simulink model "DroneDynamics_full"  (R2022b)
settings: Solver=VariableStepAuto  StartTime=0.0  StopTime=sim_time  FixedStep=dt  RelTol=1e-3
values from neighbouring files (symbols this model uses):
  b = 0.71    [Data_full.m]
  dt = 0.01    [Data_full.m]
  g_vect = [0; 0; m*g]    [Data_full.m]
  m = 3.074    [Data_full.m]
  mixer = [        -1         -1        -1         -1 ... (first row only)    [Data_full.m]
  NED2ECI = [ 1  0  0 ... (first row only)    [Data_full.m]
  omega0 = zeros(3,1)    [Data_full.m]
  p0 = zeros(3,1)    [Data_full.m]
  q0 = [1 0 0 0]'    [Data_full.m]
  tau = 1/900    (= 0.00111111111111)    [Data_full.m]
  v0 = zeros(3,1)    [Data_full.m]
undefined symbols (not defined in the file or in its folder): guidance
libraries: sharedtransform x1, simulink_extras x1, sim3dlib x1, uavsim3dlib x1
settings Model: Creator=Pietro Bruschi  LastModifiedBy=Utente
settings SFSimCC: SimCustomHeaderCode="#include \"controller_full.h\""  SimUserSources=controller_full.c  CustomCodeGlobalsAsFunctionIO=on

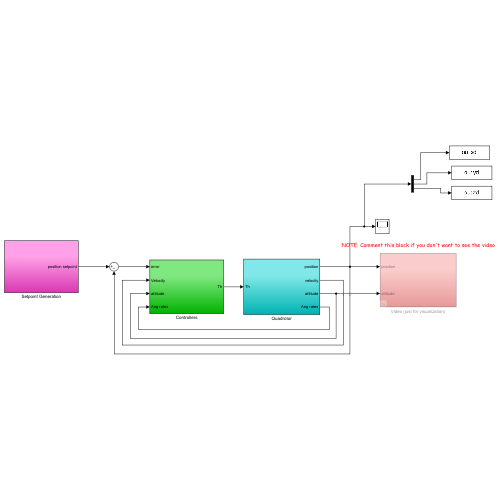
[thumbnail: Simulink's stored preview of the top-level diagram]
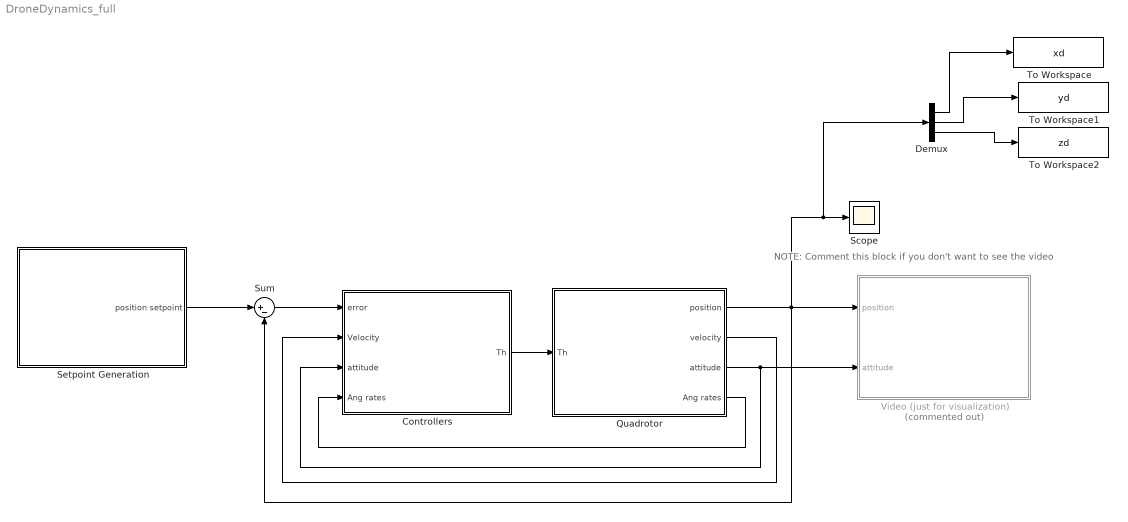
== system DroneDynamics_full ==
  note: NOTE: Comment this block if you don't want to see the video
  Controllers : Subsystem
  Demux : Demux  Outputs=3
  Quadrotor : Subsystem
  Scope : Scope
  Setpoint Generation : Subsystem
  Sum : Sum  Inputs=|+-
  To Workspace : ToWorkspace  VariableName=xd  SampleTime=-1
  To Workspace1 : ToWorkspace  VariableName=yd  SampleTime=-1
  To Workspace2 : ToWorkspace  VariableName=zd  SampleTime=-1
  Video (just for visualization) : Subsystem  Commented=on
  wires:
  Sum/1 -> Controllers/1("error ")
  Controllers/1(Th) -> Quadrotor/1(Th)
  Quadrotor/1(position) -> Demux/1, Scope/1, Sum/2, Video (just for visualization)/1(position)
  Setpoint Generation/1(position setpoint) -> Sum/1
  Quadrotor/4(Ang rates) -> Controllers/4(Ang rates)
  Quadrotor/3(attitude) -> Controllers/3(attitude), Video (just for visualization)/2(attitude)
  Quadrotor/2(velocity) -> Controllers/2(Velocity)
  Demux/1 -> To Workspace/1
  Demux/3 -> To Workspace2/1
  Demux/2 -> To Workspace1/1

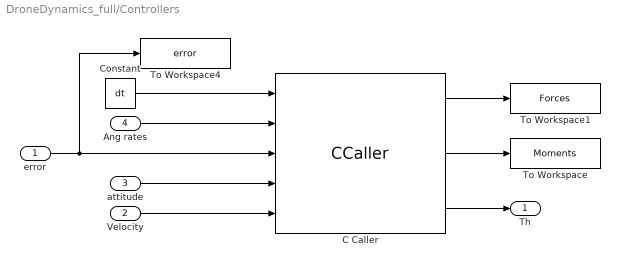
== system DroneDynamics_full/Controllers ==
  "error " : Inport
  Velocity : Inport  Port=2
  attitude : Inport  Port=3
  Ang rates : Inport  Port=4
  C Caller : CCaller  FunctionName=loop  PortSpecificationStruct="%)30     .    .!8   8    (     @         %    \"     T    !     0         %  0 \"0    $    _    07)G3F%M90  4&]R=$YA;64 4V-O<&4     26YD97@     5'EP90      4VEZ90      27-';&]B86P   X    X    !@    @    $          4    (     0    8    !         !     &    1%]L87-T   .    .     8    (    !          %    \"     $    &     0         0    !@   $1?;&%S=   #@   #@    &    \"     0         !0    @    !   ...(+7287 chars)"  SampleTime=dt
  Constant : Constant  Value=dt
  To Workspace : ToWorkspace  VariableName=Moments  SaveFormat=Timeseries  SampleTime=-1
  To Workspace1 : ToWorkspace  VariableName=Forces  SaveFormat=Timeseries  SampleTime=-1
  To Workspace4 : ToWorkspace  VariableName=error  SaveFormat=Timeseries  SampleTime=-1
  Th : Outport
  wires:
  "error "/1 -> To Workspace4/1, C Caller/3
  C Caller/1 -> To Workspace1/1
  C Caller/2 -> To Workspace/1
  C Caller/3 -> Th/1
  Velocity/1 -> C Caller/5
  attitude/1 -> C Caller/4
  Ang rates/1 -> C Caller/2
  Constant/1 -> C Caller/1

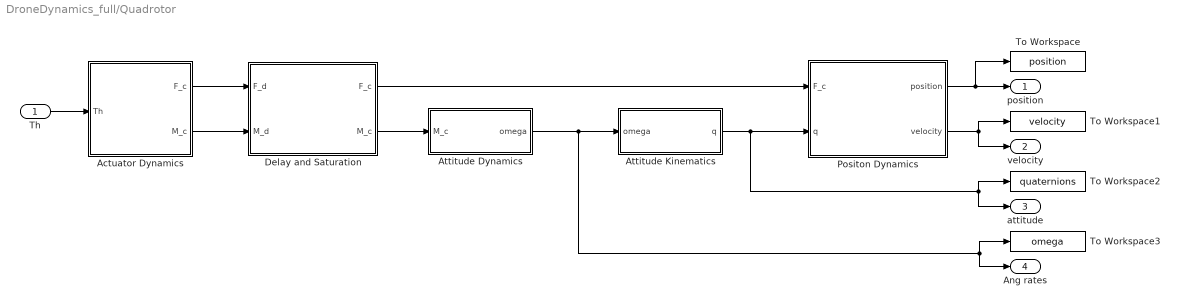
== system DroneDynamics_full/Quadrotor ==
  Th : Inport
  Actuator Dynamics : Subsystem
  Attitude Dynamics : Subsystem
  Attitude Kinematics : Subsystem
  Delay and Saturation : Subsystem
  Positon Dynamics : Subsystem
  To Workspace : ToWorkspace  VariableName=position  SaveFormat=Timeseries  SampleTime=-1
  To Workspace1 : ToWorkspace  VariableName=velocity  SaveFormat=Timeseries  SampleTime=-1
  To Workspace2 : ToWorkspace  VariableName=quaternions  SaveFormat=Timeseries  SampleTime=-1
  To Workspace3 : ToWorkspace  VariableName=omega  SaveFormat=Timeseries  SampleTime=-1
  position : Outport
  velocity : Outport  Port=2
  attitude : Outport  Port=3
  Ang rates : Outport  Port=4
  wires:
  Attitude Dynamics/1(omega) -> To Workspace3/1, Ang rates/1, Attitude Kinematics/1(omega)
  Attitude Kinematics/1(q) -> To Workspace2/1, attitude/1, Positon Dynamics/2(q)
  Positon Dynamics/1(position) -> To Workspace/1, position/1
  Positon Dynamics/2(velocity) -> velocity/1, To Workspace1/1
  Th/1 -> Actuator Dynamics/1(Th)
  Delay and Saturation/2(M_c) -> Attitude Dynamics/1(M_c)
  Actuator Dynamics/2(M_c) -> Delay and Saturation/2(M_d)
  Actuator Dynamics/1(F_c) -> Delay and Saturation/1(F_d)
  Delay and Saturation/1(F_c) -> Positon Dynamics/1(F_c)

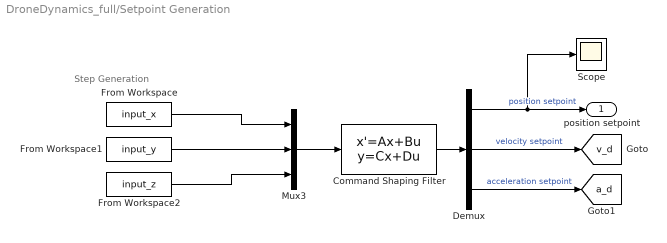
== system DroneDynamics_full/Setpoint Generation ==
  note: Step Generation
  "Command Shaping Filter " : StateSpace  A=guidance.A_d  B=guidance.B_d  C=eye(9)  D=zeros(9,3)  InitialCondition=zeros(9,1)  ParameterTunability=Unconstrained
  Demux : Demux  Outputs=3
  From Workspace : FromWorkspace  VariableName=input_x
  From Workspace1 : FromWorkspace  VariableName=input_y
  From Workspace2 : FromWorkspace  VariableName=input_z
  Mux3 : Mux  Inputs=3
  Scope : Scope
  position setpoint : Outport
  tag scope: a_d=global, v_d=global
  wires:
  "Command Shaping Filter "/1 -> Demux/1
  Mux3/1 -> "Command Shaping Filter "/1
  Demux/2 -> [v_d]  "velocity setpoint"
  Demux/3 -> [a_d]  "acceleration setpoint"
  Demux/1 -> Scope/1, position setpoint/1  "position setpoint"
  From Workspace/1 -> Mux3/1
  From Workspace1/1 -> Mux3/2
  From Workspace2/1 -> Mux3/3

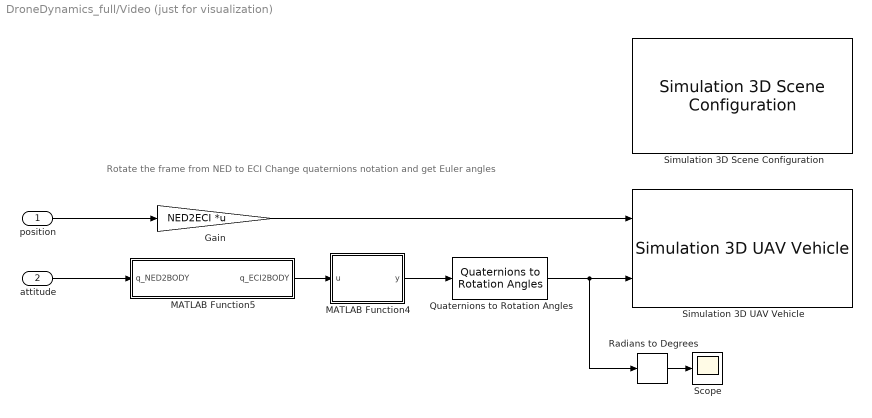
== system DroneDynamics_full/Video (just for visualization) ==
  note: Rotate the frame from NED to ECI
      | Change quaternions notation and get Euler angles
  position : Inport
  attitude : Inport  Port=2
  Gain : Gain  Gain=NED2ECI  Multiplication=Matrix(K*u)
  MATLAB Function4 : MATLAB Function  TreatAsAtomicUnit=on
  MATLAB Function5 : MATLAB Function  TreatAsAtomicUnit=on
  Quaternions to Rotation Angles : sharedtransform/Quaternions to Rotation Angles  rotationOrder=ZYX  aMode=aMode
  Radians to Degrees : simulink_extras/Transformations/Radians to Degrees
  Scope : Scope
  Simulation 3D Scene Configuration : sim3dlib/Simulation 3D Scene Configuration  Priority=0  ProjectFormat=Default Scenes  SceneDesc=US city block  ProjectName=C:\Program Files\MATLAB\R2022b\toolbox\shared\sim3d_projects\automotive_project\UE4\WindowsNoEditor\VehicleSimulation.exe  ScenePath=/Game/Maps/USCityBlock  EnableOpenDRIVE=off  vehTagList={'Scene Origin';'SimulinkVehicle1'}  vehTag=Scene Origin  OpVisEn=off  Ts=0.01  EnableWindow=on  EnableRemoteAccess=off  EnableWeather=off  SunAltitude=40.0  SunAzimuth=90  clouds=10  wind=1  fog=0  rain=0  EnableGeospatial=off  OriginHeight=200  OriginLatitude=40.744652  OriginLongitude=-73.988864  MapStyle=Aerial  AdditionalAssetIDs=[]  UseAdvancedSunSky=off  SolarTime=11  TimeZone=-5  Day=21  Month=9  Year=2022  UseDaylightSavingTime=on  DSTStartDay=10  DSTStartMonth=3  DSTEndDay=3  DSTEndMonth=11  DSTSwitchHour=2  sensorTag=MainCamera1  sensorId=1  sensorName=MainCamera1  mountLoc=Origin  offsetFlag=off  tmountOffset=[0, 0, 0]  rmountOffset=[0, 0, 0]  HorizontalResolution=1280  VerticalResolution=720  HorizontalFOV=60  mountPoint=[0 0 0]  mountOrientation=[0 0 0]  aMode=4  ID=1  GeoTrigger=Inactive
      settings: LibrarySourceBlock=uavsim3dlib/Simulation 3D Scene Configuration
  Simulation 3D UAV Vehicle : uavsim3dlib/Simulation 3D UAV Vehicle  Priority=-1  Mesh=Quadrotor  MeshPath=/MathWorksUAVContent/UAVs/HexaRotorUAV/HexaRotor.HexaRotor  Color=Black  ActorName=SimulinkVehicle1  InitialTranslation=[0 0 .2]  InitialRotation=[0 0 0]  SampleTime=-1  ActorType=SimulinkVehicle  ID=1  aMode=4  ActorTag=SimulinkVehicle1
  wires:
  Radians to Degrees/1 -> Scope/1
  MATLAB Function5/1(q_ECI2BODY) -> MATLAB Function4/1(u)
  position/1 -> Gain/1
  MATLAB Function4/1(y) -> Quaternions to Rotation Angles/1
  Gain/1 -> Simulation 3D UAV Vehicle/1
  attitude/1 -> MATLAB Function5/1(q_NED2BODY)
  Quaternions to Rotation Angles/1 -> Simulation 3D UAV Vehicle/2, Radians to Degrees/1

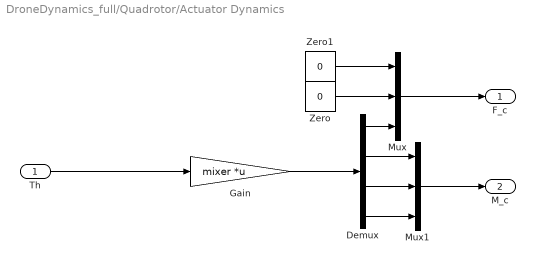
== system DroneDynamics_full/Quadrotor/Actuator Dynamics ==
  Th : Inport
  Demux : Demux
  Gain : Gain  Gain=mixer  Multiplication=Matrix(K*u) (u vector)
  Mux : Mux  Inputs=3
  Mux1 : Mux  Inputs=3
  Zero : Constant  Value=0  OutDataTypeStr=Inherit: Inherit via back propagation
  Zero1 : Constant  Value=0  OutDataTypeStr=Inherit: Inherit via back propagation
  F_c : Outport
  M_c : Outport  Port=2
  wires:
  Gain/1 -> Demux/1
  Mux/1 -> F_c/1
  Demux/1 -> Mux/3
  Zero1/1 -> Mux/1
  Zero/1 -> Mux/2
  Mux1/1 -> M_c/1
  Demux/2 -> Mux1/1
  Demux/3 -> Mux1/2
  Demux/4 -> Mux1/3
  Th/1 -> Gain/1

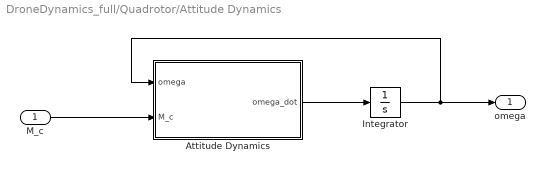
== system DroneDynamics_full/Quadrotor/Attitude Dynamics ==
  M_c : Inport
  Attitude Dynamics : MATLAB Function  TreatAsAtomicUnit=on
  Integrator : Integrator  InitialCondition=omega0
  omega : Outport
  wires:
  M_c/1 -> Attitude Dynamics/2(M_c)
  Attitude Dynamics/1(omega_dot) -> Integrator/1
  Integrator/1 -> Attitude Dynamics/1(omega), omega/1

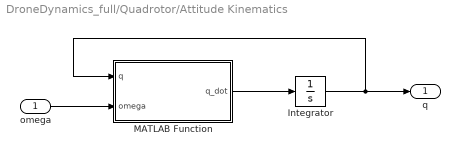
== system DroneDynamics_full/Quadrotor/Attitude Kinematics ==
  omega : Inport
  Integrator : Integrator  InitialCondition=q0
  MATLAB Function : MATLAB Function  TreatAsAtomicUnit=on
  q : Outport
  wires:
  Integrator/1 -> MATLAB Function/1(q), q/1
  omega/1 -> MATLAB Function/2(omega)
  MATLAB Function/1(q_dot) -> Integrator/1

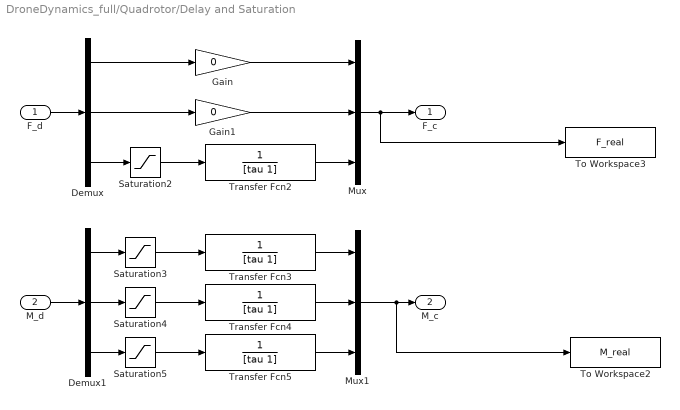
== system DroneDynamics_full/Quadrotor/Delay and Saturation ==
  F_d : Inport
  M_d : Inport  Port=2
  Demux : Demux  Outputs=3
  Demux1 : Demux  Outputs=3
  Gain : Gain  Gain=0
  Gain1 : Gain  Gain=0
  Mux : Mux  Inputs=3
  Mux1 : Mux  Inputs=3
  Saturation2 : Saturate  UpperLimit=250  LowerLimit=-250
  Saturation3 : Saturate  UpperLimit=250*b  LowerLimit=-250*b
  Saturation4 : Saturate  UpperLimit=250*b  LowerLimit=-250*b
  Saturation5 : Saturate  UpperLimit=250*b  LowerLimit=-250*b
  To Workspace2 : ToWorkspace  VariableName=M_real  SaveFormat=Timeseries  SampleTime=-1
  To Workspace3 : ToWorkspace  VariableName=F_real  SaveFormat=Timeseries  SampleTime=-1
  Transfer Fcn{2..5} (4 alike) : TransferFcn  Denominator=[tau 1]
  F_c : Outport
  M_c : Outport  Port=2
  wires:
  F_d/1 -> Demux/1
  Mux/1 -> To Workspace3/1, F_c/1
  Gain/1 -> Mux/1
  Gain1/1 -> Mux/2
  Mux1/1 -> To Workspace2/1, M_c/1
  M_d/1 -> Demux1/1
  Demux/2 -> Gain1/1
  Demux/1 -> Gain/1
  Transfer Fcn4/1 -> Mux1/2
  Transfer Fcn5/1 -> Mux1/3
  Transfer Fcn2/1 -> Mux/3
  Transfer Fcn3/1 -> Mux1/1
  Demux/3 -> Saturation2/1
  Demux1/1 -> Saturation3/1
  Demux1/2 -> Saturation4/1
  Demux1/3 -> Saturation5/1
  Saturation2/1 -> Transfer Fcn2/1
  Saturation5/1 -> Transfer Fcn5/1
  Saturation4/1 -> Transfer Fcn4/1
  Saturation3/1 -> Transfer Fcn3/1

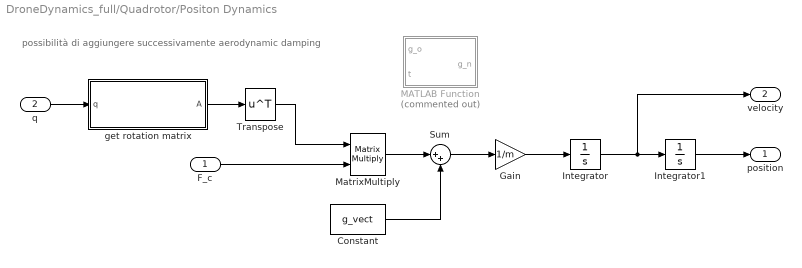
== system DroneDynamics_full/Quadrotor/Positon Dynamics ==
  note: possibilità di aggiungere successivamente aerodynamic damping
  F_c : Inport
  q : Inport  Port=2
  Constant : Constant  Value=g_vect
  Gain : Gain  Gain=1/m
  Integrator : Integrator  InitialCondition=v0
  Integrator1 : Integrator  InitialCondition=p0
  MATLAB Function : MATLAB Function  Commented=on  TreatAsAtomicUnit=on
  MatrixMultiply : Product  Multiplication=Matrix(*)
  Sum : Sum  Inputs=|++
  Transpose : Math  Operator=transpose
  get rotation matrix : MATLAB Function  TreatAsAtomicUnit=on
  position : Outport
  velocity : Outport  Port=2
  wires:
  Integrator/1 -> velocity/1, Integrator1/1
  Gain/1 -> Integrator/1
  MatrixMultiply/1 -> Sum/1
  q/1 -> get rotation matrix/1(q)
  get rotation matrix/1(A) -> Transpose/1
  Integrator1/1 -> position/1
  Sum/1 -> Gain/1
  F_c/1 -> MatrixMultiply/2
  Transpose/1 -> MatrixMultiply/1
  Constant/1 -> Sum/2

== matlab function DroneDynamics_full/Quadrotor/Attitude Dynamics/Attitude Dynamics ==
  data: omega input; omega_dot output; M_c input; Drone parameter
function omega_dot = fcn(omega, M_c, Drone)

J = Drone.J;
Jinv = Drone.Jinv;

omega_dot = Jinv * (-cross(omega,J*omega) + M_c);

== matlab function DroneDynamics_full/Quadrotor/Positon Dynamics/get rotation matrix ==
  data: q input; A output
function A = fcn(q)

q = q/norm(q);

q_v = q(1:3);

q_cross = [     0 -q(3)  q(2) ;
             q(3)     0 -q(1) ;
            -q(2)  q(1)     0 ];

A = (q(4) - q_v'*q_v)*eye(3) + 2*q_v*q_v' - 2*q(4)*q_cross;

% A = quat2dcm(q);

== matlab function DroneDynamics_full/Quadrotor/Positon Dynamics/MATLAB Function ==
  data: g_o input; g_n output; t input
function g_n = fcn(g_o,t)

g_n = g_o*(t>5);

== matlab function DroneDynamics_full/Video (just for visualization)/MATLAB Function4 ==
  data: u input; y output
function y = fcn(u)

% Convert from 1234 to 0123 notation

y = zeros(4,1);

y(1) = u(4);
y(2:4) = u(1:3);

== matlab function DroneDynamics_full/Video (just for visualization)/MATLAB Function5 ==
  data: q_NED2BODY input; q_ECI2BODY output
function q_ECI2BODY = fcn(q_NED2BODY)

% Convert quaternions from NED to ECI frames

q_ECI2NED = [ -1 0 0 0 ]';

% qv1 = [q_ECI2NED(1), q_ECI2NED(2), q_ECI2NED(3)]';
% qs1 = q_ECI2NED(4);
% 
% qv2 = [q_NED2BODY(1), q_NED2BODY(2), q_NED2BODY(3)]';
% qs2 = q_NED2BODY(4);
% 
% q_ECI2BODY = [qs1 * qv2 + qs2 * qv1 - cross( qv1, qv2 ) ;
%               qs1 * qs2 - dot( qv1, qv2 )        ];

Q = [  q_NED2BODY(4)  q_NED2BODY(3) -q_NED2BODY(2)  q_NED2BODY(1) ;
      -q_NED2BODY(3)  q_NED2BODY(4)  q_NED2BODY(1)  q_NED2BODY(2) ;
       q_NED2BODY(2) -q_NED2BODY(1)  q_NED2BODY(4)  q_NED2BODY(3) ; 
      -q_NED2BODY(1) -q_NED2BODY(2) -q_NED2BODY(3)  q_NED2BODY(4) ];

q_ECI2BODY = Q * q_ECI2NED;
q_ECI2BODY = q_ECI2BODY / norm(q_ECI2BODY);

== matlab function DroneDynamics_full/Quadrotor/Attitude Kinematics/MATLAB Function ==
  data: q input; q_dot output; omega input
function q_dot = fcn(q, omega)

q = q/norm(q);

Omega = [       0   omega(3) -omega(2) omega(1) ;
         -omega(3)        0   omega(1) omega(2) ;
          omega(2) -omega(1)        0  omega(3) ;
         -omega(1) -omega(2) -omega(3)       0  ];

q_dot = 1/2 * Omega * q;
